simulink model "Junctions1V0_tmp"  (Simulink 8.3)
settings: Solver=ode45  StartTime=0.0  StopTime=10.0  RelTol=1e-3
settings Model: Creator=scaife  LastModifiedBy=bourbouh  CovSFcnEnable=on  ExtModeAutoUpdateStatusClock=off
settings DataIOCC: SignalLoggingName=sigsOut
settings DebuggingCC: SaveWithParameterizedLinksMsg=none  SignalResolutionControl=TryResolveAllWithWarning  SolverPrmCheckMsg=none  MultiTaskDSMMsg=warning  MultiTaskCondExecSysMsg=none  FrameProcessingCompatibilityMsg=error  StateNameClashWarn=none  StrictBusMsg=None
settings HardwareCC: TargetUnknown=on
settings SFSimCC: SimParseCustomCode=off
settings GRTTargetCC: GeneratePreprocessorConditionals=Use local settings

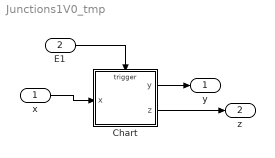
== system Junctions1V0_tmp ==
  x : Inport
  E1 : Inport  Port=2
  Chart : Stateflow chart  TreatAsAtomicUnit=on
      settings: PermitHierarchicalResolution=ParametersOnly
  y : Outport
  z : Outport  Port=2
  wires:
  Chart/1(y) -> y/1
  Chart/2(z) -> z/1
  E1/1 -> Chart/Trigger
  x/1 -> Chart/1(x)

== stateflow chart Chart ==
  state A
  state B
  state C
  B -> A : [x>3]
  (default) -> A
  C -> A : [x>3]
  A -> (junction 10) : E1[x>0]{y++}/z+=2
  (junction 10) -> C [order 2] : [x<=2]{y++}/z++
  (junction 10) -> B [order 1] : [x>2]{y+=2}/z++;z++
  data: x input int32; y output int32 =1; z output int32 =2
  events: E1 input EITHER_EDGE_EVENT
